simulink model "ThreeHarmonicCurrentInNeutralPoint"  (Simulink 7.9)
settings: Solver=ode45  StartTime=0.0  StopTime=1  MaxStep=50e-6  RelTol=1e-3
InitFcn:
  | Phi=0.5*pi;
libraries: powerlib x1
settings Model: Creator=H002220  LastModifiedBy=H002220

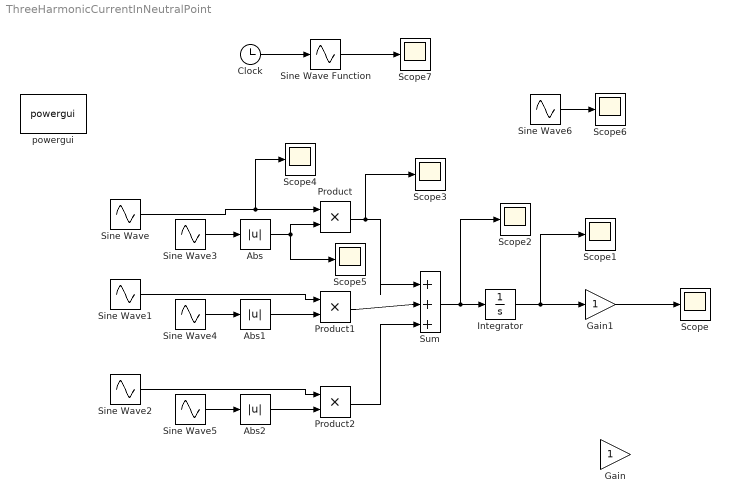
== system ThreeHarmonicCurrentInNeutralPoint ==
  Abs : Abs
  Abs1 : Abs
  Abs2 : Abs
  Clock : Clock
  Gain : Gain
  Gain1 : Gain
  Integrator : Integrator
  Product : Product  RndMeth=Zero
  Product1 : Product  RndMeth=Zero
  Product2 : Product  RndMeth=Zero
  Scope{,1..7} (8 alike) : Scope
      Scope2 settings: SaveName=ScopeData2
      Scope3 settings: SaveName=ScopeData3
      Scope4 settings: SaveName=ScopeData4
      Scope5 settings: SaveName=ScopeData5
      Scope6 settings: SaveName=ScopeData6
      Scope7 settings: SaveName=ScopeData7
  Sine Wave : Sin  Frequency=40*2*pi
  Sine Wave Function : Sin  TimeSource=Use external signal  Frequency=100*pi  SampleTime=0
  Sine Wave1 : Sin  Frequency=40*2*pi  Phase=-2*pi/3  SampleTime=0
  Sine Wave2 : Sin  Frequency=40*2*pi  Phase=2*pi/3  SampleTime=0
  Sine Wave3 : Sin  Frequency=40*2*pi  Phase=Phi  SampleTime=0
  Sine Wave4 : Sin  Frequency=40*2*pi  Phase=Phi-2*pi/3  SampleTime=0
  Sine Wave5 : Sin  Frequency=40*2*pi  Phase=Phi+2*pi/3  SampleTime=0
  Sine Wave6 : Sin  SampleTime=0
  Sum : Sum  Inputs=|+++
  powergui : powerlib/powergui  Priority=1  SimulationMode=Discrete  SolverType=Tustin  SampleTime=50e-6  frequency=60  SPID=off  DisableSnubberDevices=off  DisableRonSwitches=off  DisableVfSwitches=off  SwTol=0  Interpol=off  DisplayEquations=off  FunctionMessages=off  frequencyindice=60  Pbase=100e6  ErrMax=1e-4  Iterations=50  UnitsV=kV  UnitsW=MW  echomessages=off  HookPort=off  EnableUseOfTLC=off  x0status=blocks  RestoreLinks=warning  ResistiveCurrentMeasurement=off  Ylog=off  Xlog=on  ShowGrid=off  save=off  variable=ZData  structure=ScopeData2  ZoomFFT=off  StartTime=0.0  cycles=1  DisplayStyle=2  fundamental=120  FreqAxis=off  MaxFrequency=1000  frequencyindicesteady=1  display=off  methode=off
  wires:
  Sine Wave3/1 -> Abs/1
  Sine Wave4/1 -> Abs1/1
  Sine Wave5/1 -> Abs2/1
  Sine Wave/1 -> Product/1, Scope4/1
  Abs/1 -> Product/2, Scope5/1
  Abs1/1 -> Product1/2
  Sine Wave1/1 -> Product1/1
  Abs2/1 -> Product2/2
  Sine Wave2/1 -> Product2/1
  Product1/1 -> Sum/2
  Product/1 -> Sum/1, Scope3/1
  Product2/1 -> Sum/3
  Sum/1 -> Integrator/1, Scope2/1
  Integrator/1 -> Gain1/1, Scope1/1
  Gain1/1 -> Scope/1
  Sine Wave6/1 -> Scope6/1
  Clock/1 -> Sine Wave Function/1
  Sine Wave Function/1 -> Scope7/1
